simulink model "DE_1ex"  (Simulink 9.1)
settings: Solver=VariableStepAuto  StartTime=0.0  StopTime=0.4  RelTol=1e-3  AbsTol=1e-6
libraries: elements x1, simulink x1
settings Model: Creator=PC  LastModifiedBy=renji  ExtModeTrigMode=oneshot  ExtModeArmWhenConnect=off
settings SolverCC: AutoScaleAbsTol=off
settings DataIOCC: SignalLoggingSaveFormat=ModelDataLogs
settings OptimizationCC: BlockReduction=off  BooleanDataType=off
settings DebuggingCC: SaveWithParameterizedLinksMsg=none  SignalResolutionControl=TryResolveAllWithWarning  MultiTaskDSMMsg=warning  MultiTaskCondExecSysMsg=none
settings HardwareCC: TargetUnknown=on
settings GRTTargetCC: GeneratePreprocessorConditionals=Disable all

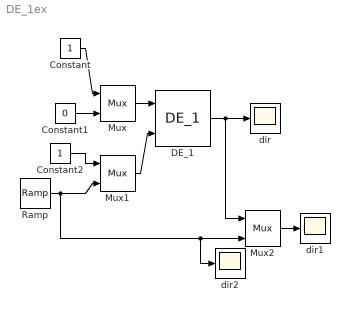
== system DE_1ex ==
  "  DE_1" : elements/  DE_1  alpha=10  beta=170  fs=20*60
  Constant : Constant
  Constant1 : Constant  Value=0
  Constant2 : Constant
  Mux : Mux  Inputs=2
  Mux1 : Mux  Inputs=2
  Mux2 : Mux  Inputs=2
  Ramp : simulink/Sources/Ramp  slope=1000  start=0  InitialOutput=0
  dir : Scope
  dir1 : Scope
  dir2 : Scope
  wires:
  Mux/1 -> "  DE_1"/1
  Constant1/1 -> Mux/2
  Constant/1 -> Mux/1
  Mux1/1 -> "  DE_1"/2
  Constant2/1 -> Mux1/1
  Mux2/1 -> dir1/1
  "  DE_1"/1 -> dir/1, Mux2/1
  Ramp/1 -> Mux1/2, Mux2/2, dir2/1
